simulink model "DiscreteImplementationContinuousController"  (Simulink 8.8)
settings: Solver=ode45  StartTime=0.0  StopTime=50  FixedStep=Ts  MaxStep=Ts  RelTol=1e-3  EnableMultiTasking=on
PostLoadFcn:
  | , if any(exist('dsrtsu_mdlpostloadfcn', 'file') == [2, 3, 6]), try dsrtsu_mdlpostloadfcn('Execute', bdroot); catch fprintf('Error in PostLoadFcn (dsrtsu_mdlpostloadfcn) for model "%s":\n %s\n', bdroot, lasterr); end, end,
values from neighbouring files (symbols this model uses):
  C_den = [1 12000 21360000 13600000000]    [Assignment4.mat]    (also in Assignment4bu.mat = [1 13157 43251540]; assignment4.m = den(1:end-1); assignment6.m = C_den(1:end-1))
  C_num = [0 0 272000000000 68054400000000 13600000000000]    [Assignment4.mat]    (also in Assignment4bu.mat = [0 12801000000 2715476130000 43668537738000]; assignment4.m = num)
  I0 = 2.36    [Assignment3.mat]    (also in assignment3.m = I(2))
  Ts = 1/2000    (= 0.0005)    [assignment5.m]    (also in assignment6.m = 0.002)
  Y0 = 0.049    [Assignment3.mat]    (also in assignment3.m = Y(2))
undefined symbols (not defined in the file or in its folder): Cd_den, Cd_num, DiscIntNeverNeededParam, P_den, P_num
settings Model: DSRTSU_INTERNAL_RTI_VER=350  DSRTSU_INTERNAL_RTI_TYPE=rti1104  Creator=whendrix  LastModifiedBy=s143065
settings OptimizationCC: BlockReduction=off  OptimizeBlockIOStorage=off  BufferReuse=off  GlobalBufferReuse=off  ExpressionFolding=off  ExpressionDepthLimit=2147483647  LocalBlockOutputs=off
settings DebuggingCC: SolverPrmCheckMsg=warning
settings HardwareCC: ProdIntDivRoundTo=Zero  ProdEndianess=BigEndian  ProdHWDeviceType=Generic->Custom  TargetIntDivRoundTo=Zero  TargetEndianess=BigEndian  TargetHWDeviceType=Generic->Custom
settings RTWCC: SystemTargetFile=rti1104.tlc  MakeCommand=make_rti  TemplateMakefile=rti1104.tmf  Description=dSPACE DS1104 Hardware Platform
settings STFCustomTargetCC: MatFileLogging=on  CPPClassGenCompliant=on  SystemTargetFile=rti1104.tlc
settings GRTTargetCC: ParMdlRefBuildCompliant=off  CompOptLevelCompliant=off  ConcurrentExecutionCompliant=off  GeneratePreprocessorConditionals=Use local settings  UseToolchainInfoCompliant=off  ExtModeMexFile=noextcomm
settings CustomProperty: DataType=RTWOptions_EnumType_C__dSPACE6p5_matlab_rti1104_tlc_rti1104_1InitialSimState  Value=RUN
settings EnumStrPairs: String=RUN

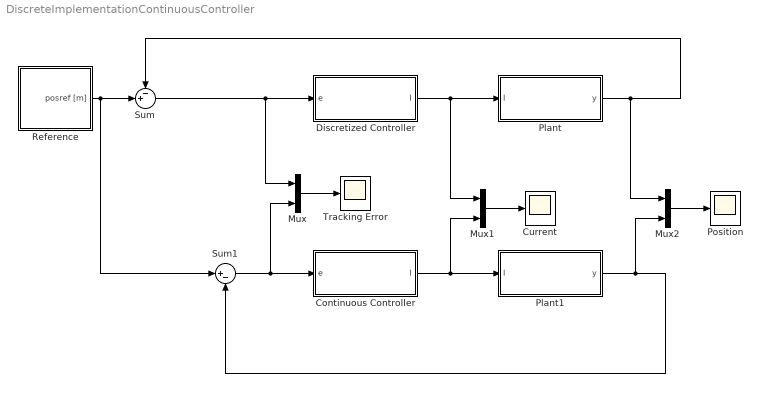
== system DiscreteImplementationContinuousController ==
  Continuous Controller : Subsystem
  Current : Scope
  Discretized Controller : Subsystem
  Mux : Mux  Inputs=2
  Mux1 : Mux  Inputs=2
  Mux2 : Mux  Inputs=2
  Plant : Subsystem
  Plant1 : Subsystem
  Position : Scope
  Reference : Subsystem
  Sum : Sum  Inputs=-+|
  Sum1 : Sum  Inputs=|+-
  Tracking Error : Scope
  wires:
  Sum/1 -> Mux/1, Discretized Controller/1(e)
  Discretized Controller/1(I) -> Plant/1(I), Mux1/1
  Reference/1(posref [m]) -> Sum1/1, Sum/2
  Sum1/1 -> Mux/2, Continuous Controller/1(e)
  Continuous Controller/1(I) -> Plant1/1(I), Mux1/2
  Plant1/1(y) -> Sum1/2, Mux2/2
  Mux/1 -> Tracking Error/1
  Plant/1(y) -> Sum/1, Mux2/1
  Mux1/1 -> Current/1
  Mux2/1 -> Position/1

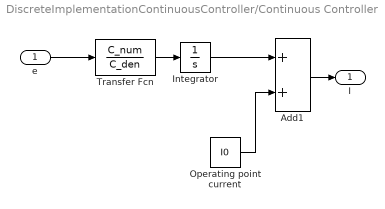
== system DiscreteImplementationContinuousController/Continuous Controller ==
  e : Inport
  Add1 : Sum
  Integrator : Integrator  LimitOutput=on  UpperSaturationLimit=3-I0  LowerSaturationLimit=-I0
  Operating point current : Constant  Value=I0
  Transfer Fcn : TransferFcn  Numerator=C_num  Denominator=C_den
  I : Outport
  wires:
  e/1 -> Transfer Fcn/1
  Operating point current/1 -> Add1/2
  Transfer Fcn/1 -> Integrator/1
  Add1/1 -> I/1
  Integrator/1 -> Add1/1

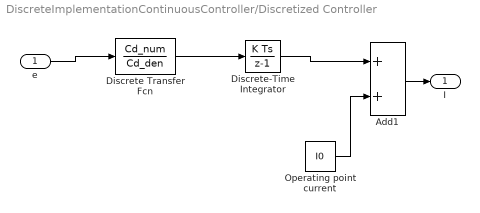
== system DiscreteImplementationContinuousController/Discretized Controller ==
  e : Inport
  Add1 : Sum
  Discrete Transfer Fcn : DiscreteTransferFcn  Numerator=Cd_num  Denominator=Cd_den  SampleTime=Ts
  Discrete-Time Integrator : DiscreteIntegrator  gainval=1/Ts  SampleTime=Ts  LimitOutput=on  UpperSaturationLimit=3-I0  LowerSaturationLimit=-I0  ICPrevOutput=DiscIntNeverNeededParam  ICPrevScaledInput=DiscIntNeverNeededParam
  Operating point current : Constant  Value=I0
  I : Outport
  wires:
  Operating point current/1 -> Add1/2
  Discrete-Time Integrator/1 -> Add1/1
  Add1/1 -> I/1
  Discrete Transfer Fcn/1 -> Discrete-Time Integrator/1
  e/1 -> Discrete Transfer Fcn/1

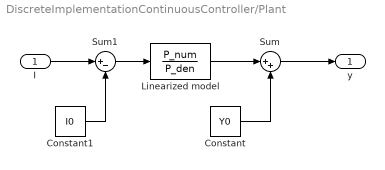
== system DiscreteImplementationContinuousController/Plant ==
  I : Inport
  Constant : Constant  Value=Y0
  Constant1 : Constant  Value=I0
  Linearized model : TransferFcn  Numerator=P_num  Denominator=P_den
  Sum : Sum  Inputs=|++
  Sum1 : Sum  Inputs=|+-
  y : Outport
  wires:
  Linearized model/1 -> Sum/1
  Sum/1 -> y/1
  Constant/1 -> Sum/2
  Sum1/1 -> Linearized model/1
  Constant1/1 -> Sum1/2
  I/1 -> Sum1/1

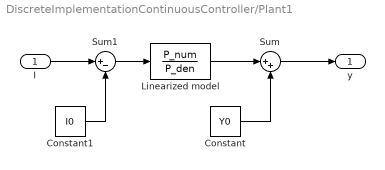
== system DiscreteImplementationContinuousController/Plant1 ==
  I : Inport
  Constant : Constant  Value=Y0
  Constant1 : Constant  Value=I0
  Linearized model : TransferFcn  Numerator=P_num  Denominator=P_den
  Sum : Sum  Inputs=|++
  Sum1 : Sum  Inputs=|+-
  y : Outport
  wires:
  Linearized model/1 -> Sum/1
  Sum/1 -> y/1
  Constant/1 -> Sum/2
  Sum1/1 -> Linearized model/1
  Constant1/1 -> Sum1/2
  I/1 -> Sum1/1

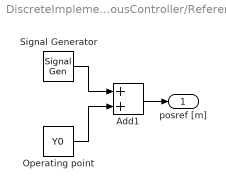
== system DiscreteImplementationContinuousController/Reference ==
  Add1 : Sum
  Operating point : Constant  Value=Y0
  Signal Generator : SignalGenerator  Amplitude=0.001
  posref [m] : Outport
  wires:
  Signal Generator/1 -> Add1/1
  Add1/1 -> posref [m]/1
  Operating point/1 -> Add1/2
